simulink model "LQG"  (R2022b)
settings: Solver=VariableStepAuto  StartTime=0.0  StopTime=40  RelTol=1e-3
values from neighbouring files (symbols this model uses):
  AA = [0 1; g/L 0]    [simConstants.m]
  BB = [0; -1/L]    [simConstants.m]
  CC = [1 0]    [simConstants.m]
  F = lqr(A,B,Q,R)    [simConstants.m]
  K = W * CC' / V2    [simConstants.m]
  Td = 100e-6    (= 0.0001)    [simConstants.m]
  Ts = 1e-3    (= 0.001)    [simConstants.m]
libraries: simulink_extras x1
settings Model: Creator=logan  LastModifiedBy=logan
settings DebuggingCC: UnconnectedInputMsg=warning  UnconnectedOutputMsg=warning  UnconnectedLineMsg=warning
settings ModelReferenceCC: EnableRefExpFcnMdlSchedulingChecks=on
settings RTWCC: DLArmComputeVersion=19.05

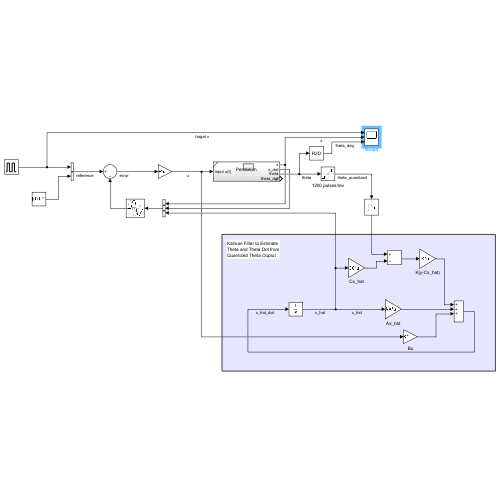
[thumbnail: Simulink's stored preview of the top-level diagram]
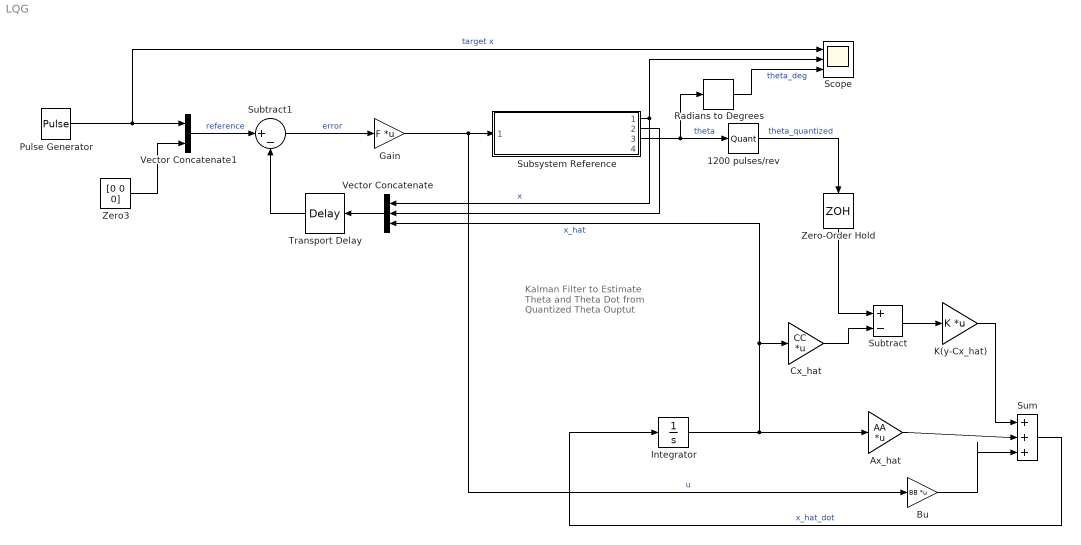
== system LQG ==
  note: Kalman Filter to Estimate
      | Theta and Theta Dot from
      | Quantized Theta Ouptut
  1200 pulses/rev : Quantizer  QuantizationInterval=(2*pi)/1200
  Ax_hat : Gain  Gain=AA  Multiplication=Matrix(K*u)
  Bu : Gain  Gain=BB  Multiplication=Matrix(K*u)
  Cx_hat : Gain  Gain=CC  Multiplication=Matrix(K*u)
  Gain : Gain  Gain=F  Multiplication=Matrix(K*u)
  Integrator : Integrator
  K(y-Cx_hat) : Gain  Gain=K  Multiplication=Matrix(K*u)
  Pulse Generator : DiscretePulseGenerator  PulseType=Time based  Period=20  PulseWidth=50
  Radians to Degrees : simulink_extras/Transformations/Radians to Degrees
  Scope : Scope  NumInputPorts=3
  Subsystem Reference : Subsystem  ReferencedSubsystem=Pendulum
  Subtract : Sum  Inputs=+-
  Subtract1 : Sum  Inputs=|+-
  Sum : Sum  Inputs=+++|
  Transport Delay : TransportDelay  DelayTime=Td*10  InitialOutput=[0 0 0 0]
  Vector Concatenate : Concatenate  NumInputs=3
  Vector Concatenate1 : Concatenate
  Zero-Order Hold : ZeroOrderHold  SampleTime=Ts
  Zero3 : Constant  Value=[0 0 0]  OutDataTypeStr=Inherit: Inherit via back propagation
  wires:
  Bu/1 -> Sum/3
  K(y-Cx_hat)/1 -> Sum/1
  Integrator/1 -> Ax_hat/1, Vector Concatenate/3, Cx_hat/1  "x_hat"
  Subtract1/1 -> Gain/1  "error"
  Gain/1 -> Bu/1, Subsystem Reference/1  "u"
  Sum/1 -> Integrator/1  "x_hat_dot"
  Subtract/1 -> K(y-Cx_hat)/1
  Cx_hat/1 -> Subtract/2
  Ax_hat/1 -> Sum/2
  Subsystem Reference/3 -> Radians to Degrees/1, 1200 pulses/rev/1  "theta"
  Subsystem Reference/1 -> Scope/2, Vector Concatenate/1  "x"
  Subsystem Reference/2 -> Vector Concatenate/2
  Radians to Degrees/1 -> Scope/3  "theta_deg"
  Zero3/1 -> Vector Concatenate1/2
  Vector Concatenate1/1 -> Subtract1/1  "reference"
  Pulse Generator/1 -> Scope/1, Vector Concatenate1/1  "target x"
  Vector Concatenate/1 -> Transport Delay/1
  Transport Delay/1 -> Subtract1/2
  1200 pulses/rev/1 -> Zero-Order Hold/1  "theta_quantized"
  Zero-Order Hold/1 -> Subtract/1
